simulink model "inversedynamicstest"  (R2025b)
settings: Solver=FixedStepAuto  StartTime=0.0  StopTime=10.0  RelTol=1e-3
settings Model: Creator=axel  LastModifiedBy=axel

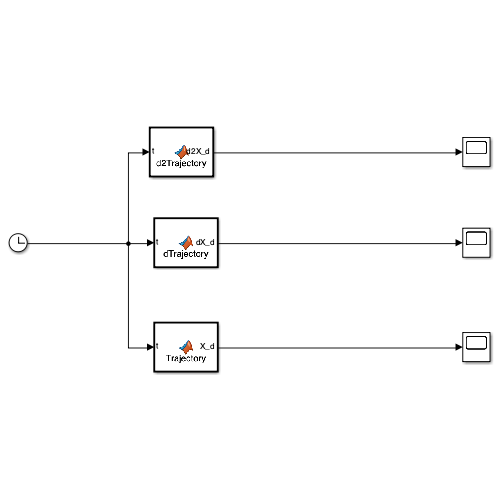
[thumbnail: Simulink's stored preview of the top-level diagram]
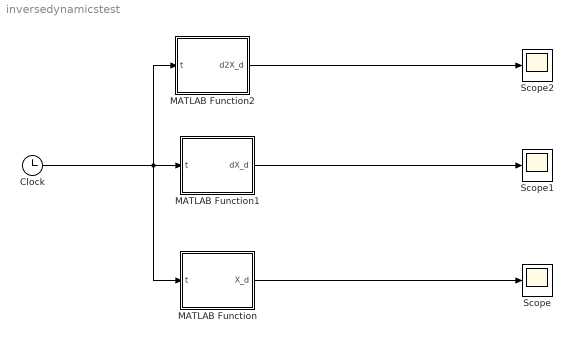
== system inversedynamicstest ==
  Clock : Clock
  MATLAB Function : MATLAB Function  TreatAsAtomicUnit=on
  MATLAB Function1 : MATLAB Function  TreatAsAtomicUnit=on
  MATLAB Function2 : MATLAB Function  TreatAsAtomicUnit=on
  Scope : Scope
      settings: ActiveDisplayYMinimum=-3.2434825756112926  ActiveDisplayYMaximum=2.3507818513540149
  Scope1 : Scope
      settings: ActiveDisplayYMinimum=-0.29462594234561307  ActiveDisplayYMaximum=0.37423794281632367
  Scope2 : Scope
      settings: ActiveDisplayYMinimum=-0.11814101984810077  ActiveDisplayYMaximum=0.11814101984810108  DataLoggingVariableName=ScopeData2
  wires:
  Clock/1 -> MATLAB Function/1(t), MATLAB Function1/1(t), MATLAB Function2/1(t)
  MATLAB Function/1(X_d) -> Scope/1
  MATLAB Function1/1(dX_d) -> Scope1/1
  MATLAB Function2/1(d2X_d) -> Scope2/1

== matlab function inversedynamicstest/MATLAB Function1 ==
  data: t input; dX_d output; dimensions parameter size=1
function dX_d = dTrajectory(t, dimensions)

coder.extrinsic('evalin', 'dX_d');
    
% Get the function handle 'f' from the MATLAB base workspace
F = evalin('base', 'dX_d'); 

% Execute the function handle
dX_d = zeros(dimensions, 1); % Initialize output for type propagation
dX_d = feval(F, t);

== matlab function inversedynamicstest/MATLAB Function ==
  data: t input; X_d output; dimensions parameter size=1
function X_d = Trajectory(t, dimensions)

coder.extrinsic('evalin', 'X_d');
    
% Get the function handle 'f' from the MATLAB base workspace
F = evalin('base', 'X_d'); 

% Execute the function handle
X_d = zeros(dimensions, 1); % Initialize output for type propagation
X_d = feval(F, t);

== matlab function inversedynamicstest/MATLAB Function2 ==
  data: t input; d2X_d output; dimensions parameter size=1
function d2X_d = d2Trajectory(t, dimensions)

coder.extrinsic('evalin', 'd2X_d');
    
% Get the function handle 'f' from the MATLAB base workspace
F = evalin('base', 'd2X_d'); 

% Execute the function handle
d2X_d = zeros(dimensions, 1); % Initialize output for type propagation
d2X_d = feval(F, t);
